simulink model "AngleConversion"  (Simulink 10.3)
settings: Solver=FixedStepAuto  StartTime=0.0  StopTime=79  FixedStep=0.02  RelTol=1e-3
settings Model: Creator=Syed Imtiaz Ali Shah  LastModifiedBy=NRPU  MultithreadedSim=on
settings DataIOCC: SaveFormat=Dataset  SignalLoggingSaveFormat=Dataset
settings OptimizationCC: ExpressionDepthLimit=128  LifeSpan=auto
settings DebuggingCC: UnderspecifiedInitializationDetection=Simplified  MergeDetectMultiDrivingBlocksExec=error  FcnCallInpInsideContextMsg=error  StateNameClashWarn=none  SFUnexpectedBacktrackingDiag=error  SFNoUnconditionalDefaultTransitionDiag=error  SFExecutionAtInitializationDiag=warning
settings HardwareCC: ProdBitPerPointer=64  ProdBitPerSizeT=64  ProdBitPerPtrDiffT=64  ProdLargestAtomicFloat=Float  ProdIntDivRoundTo=Zero  ProdEndianess=LittleEndian  ProdWordSize=64  ProdHWDeviceType=Intel->x86-64 (Windows64)
settings ModelReferenceCC: PropagateSignalLabelsOutOfModel=on
settings SFSimCC: SimCustomHeaderCode="#include \"AngleCorrection.h\""  SimUserSources=AngleCorrection.c  SimUseLocalCustomCode=on  SimAnalyzeCustomCode=on  CustomCodeGlobalsAsFunctionIO=on  DefaultCustomCodeDeterministicFunctions=All
settings RTWCC: RTWUseLocalCustomCode=on  RTWUseSimCustomCode=on  CustomHeaderCode="#include \"AngleCorrection.h\""  CustomSource=AngleCorrection.c
settings CodeAppCC: StateflowObjectComments=off
settings GRTTargetCC: TargetLangStandard=C99 (ISO)  CombineOutputUpdateFcns=on  GRTInterface=off
settings ConfigComp: CovMetricSettings=dwe  CovSaveCumulativeToWorkspaceVar=off  CovSaveSingleToWorkspaceVar=off  CovExternalEMLEnable=on

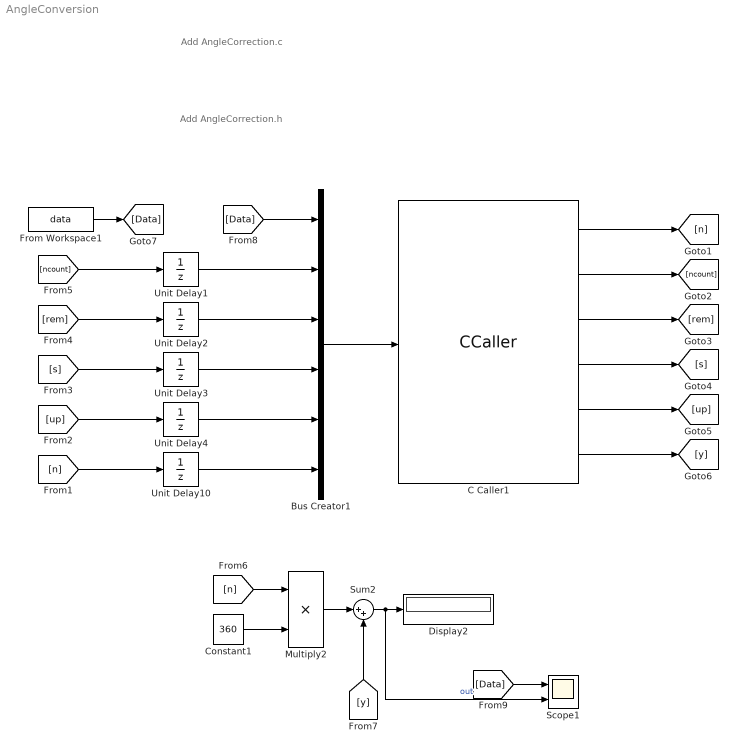
== system AngleConversion ==
  note: Add AngleCorrection.c
  note: Add AngleCorrection.h
  Bus Creator1 : BusCreator  Inputs=6
  C Caller1 : CCaller  FunctionName=fcn  PortSpecificationStruct="%)30     .    $ P   8    (     @         %    \"     <    !     0         %  0 \"0    $    _    07)G3F%M90  4&]R=$YA;64 4V-O<&4     26YD97@     5'EP90      4VEZ90      27-';&]B86P   X   !     !@    @    $          4    (     0    D    !         !     )    9&%T87-T;W)Y          X   !     !@    @    $          4    (     0    D    !         !     )    9&%T87-T;W)Y          X    X    !@    @    $     ...(+3781 chars)"
  Constant1 : Constant  Value=360
  Display2 : Display
  From Workspace1 : FromWorkspace  VariableName=data
  Multiply2 : Product
  Scope1 : Scope  NumInputPorts=2
  Sum2 : Sum  Inputs=|++
  Unit Delay{1..4,10} (5 alike) : UnitDelay  SampleTime=-1  HasFrameUpgradeWarning=on
  wires:
  C Caller1/1 -> [n]
  C Caller1/2 -> [ncount]
  C Caller1/3 -> [rem]
  C Caller1/4 -> [s]
  C Caller1/5 -> [up]
  C Caller1/6 -> [y]
  Bus Creator1/1 -> C Caller1/1
  [ncount] -> Unit Delay1/1
  Unit Delay1/1 -> Bus Creator1/2
  [rem] -> Unit Delay2/1
  Unit Delay2/1 -> Bus Creator1/3
  [s] -> Unit Delay3/1
  Unit Delay3/1 -> Bus Creator1/4
  [up] -> Unit Delay4/1
  Unit Delay4/1 -> Bus Creator1/5
  [n] -> Unit Delay10/1
  Unit Delay10/1 -> Bus Creator1/6
  Multiply2/1 -> Sum2/1
  Constant1/1 -> Multiply2/2
  Sum2/1 -> Display2/1, Scope1/2  "out"
  [n] -> Multiply2/1
  [y] -> Sum2/2
  From Workspace1/1 -> [Data]
  [Data] -> Bus Creator1/1
  [Data] -> Scope1/1
